simulink model "CC3"  (Simulink 7.5)
settings: Solver=ode45  StartTime=0.0  StopTime=300  RelTol=1e-3
settings Model: Creator=Fer  LastModifiedBy=Fer

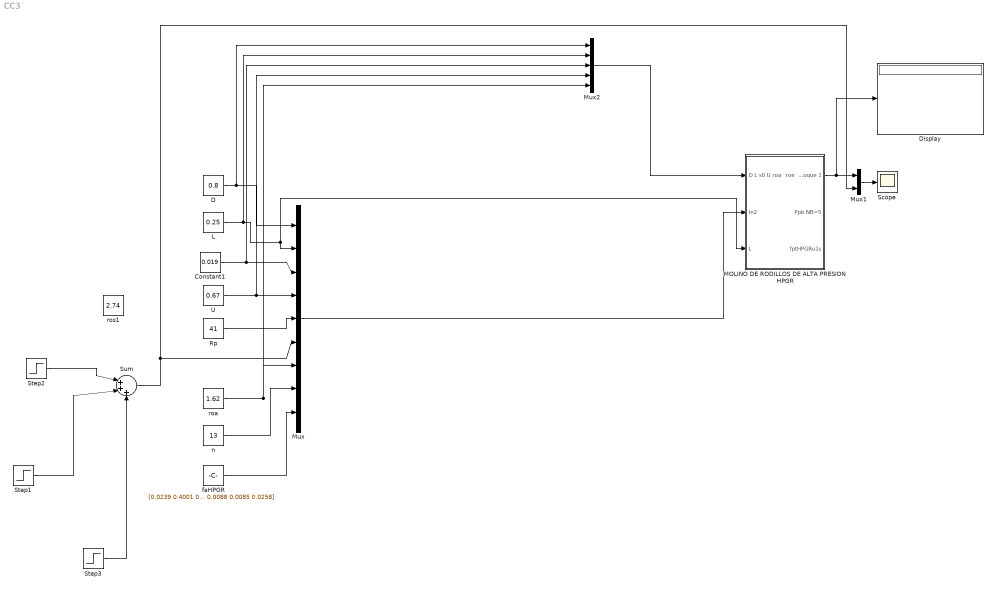
== system CC3 ==
  Constant1 : Constant  Value=0.019  OutDataType=fixdt(1, 16)  OutScaling=2^0
  D : Constant  Value=0.8  OutDataType=fixdt(1, 16)  OutScaling=2^0
  Display : Display
  L : Constant  Value=0.25  OutDataType=fixdt(1, 16)  OutScaling=2^0
  MOLINO DE RODILLOS DE ALTA PRESION HPGR : Subsystem
  Mux : Mux  Inputs=9
  Mux1 : Mux  Inputs=2
  Mux2 : Mux  Inputs=5
  Rp : Constant  Value=41  OutDataType=fixdt(1, 16)  OutScaling=2^0
  Scope : Scope
      settings: TimeRange=400  YMin=0  YMax=3  SaveName=ScopeData2
  Step1 : Step  Time=80  Before=3  After=7  SampleTime=0
  Step2 : Step  Time=80  Before=2.74  After=3  SampleTime=0
  Step3 : Step  Time=130  Before=3  SampleTime=0
  Sum : Sum  Inputs=|+++  OutDataType=fixdt(1, 16)  OutScaling=2^0
  U : Constant  Value=0.67  OutDataType=fixdt(1, 16)  OutScaling=2^0
  faHPGR : Constant  Value=[0.0239 0.4001 0.2089 0.1090 0.0549 0.0441 0.0542 0.0374 0.0159 0.0085 0.0088 0.0085 0.0258]  OutDataType=fixdt(1, 16)  OutScaling=2^0
  n : Constant  Value=13  OutDataType=fixdt(1, 16)  OutScaling=2^0
  roa : Constant  Value=1.62  OutDataType=fixdt(1, 16)  OutScaling=2^0
  ros1 : Constant  Value=2.74  OutDataType=fixdt(1, 16)  OutScaling=2^0
  wires:
  D/1 -> Mux/1, Mux2/1
  L/1 -> Mux/2, MOLINO DE RODILLOS DE ALTA PRESION HPGR/3(L), Mux2/2
  roa/1 -> Mux/7, Mux2/5
  n/1 -> Mux/8
  Mux/1 -> MOLINO DE RODILLOS DE ALTA PRESION HPGR/2(In2)
  Mux2/1 -> MOLINO DE RODILLOS DE ALTA PRESION HPGR/1(D L s0 U roa)
  faHPGR/1 -> Mux/9
  MOLINO DE RODILLOS DE ALTA PRESION HPGR/1(roe  bloque 1) -> Mux1/1, Display/1
  Mux1/1 -> Scope/1
  Step2/1 -> Sum/1
  Sum/1 -> Mux1/2, Mux/6
  Rp/1 -> Mux/5
  U/1 -> Mux/4, Mux2/4
  Step1/1 -> Sum/2
  Step3/1 -> Sum/3
  Constant1/1 -> Mux/3, Mux2/3

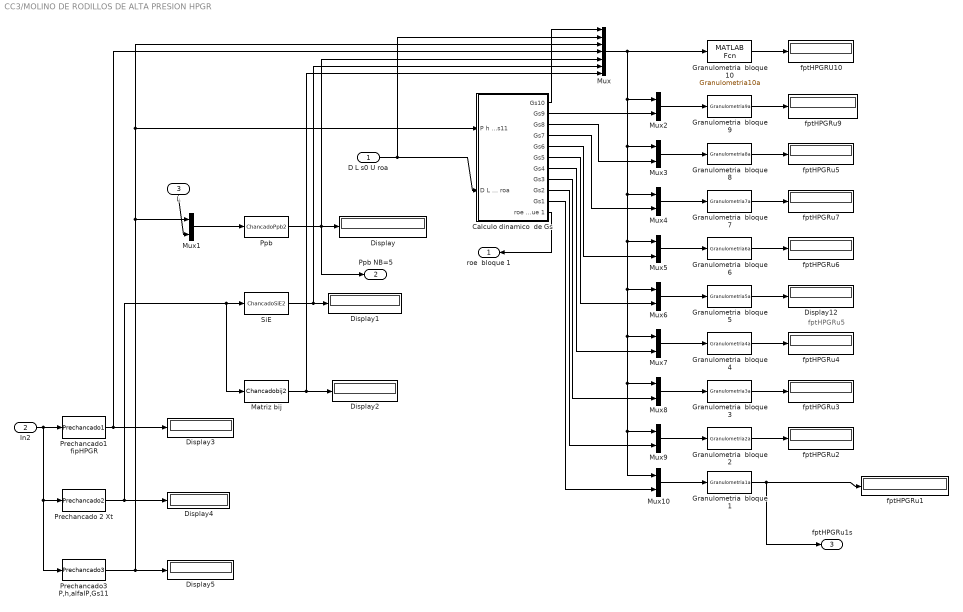
== system CC3/MOLINO DE RODILLOS DE ALTA PRESION HPGR ==
  note: fptHPGRu5
  D L s0 U roa : Inport
  In2 : Inport  Port=2
  L : Inport  Port=3
  Calculo dinamico  de Gs : Subsystem
  Display{,1..5,12} (7 alike) : Display
  Granulometria  bloque 1 : MATLABFcn  MATLABFcn=Granulometria1a
  Granulometria  bloque 10 : MATLABFcn  MATLABFcn=Granulometria10a
  Granulometria  bloque 2 : MATLABFcn  MATLABFcn=Granulometria2a
  Granulometria  bloque 3 : MATLABFcn  MATLABFcn=Granulometria3a
  Granulometria  bloque 4 : MATLABFcn  MATLABFcn=Granulometria4a
  Granulometria  bloque 5 : MATLABFcn  MATLABFcn=Granulometria5a
  Granulometria  bloque 6 : MATLABFcn  MATLABFcn=Granulometria6a
  Granulometria  bloque 7 : MATLABFcn  MATLABFcn=Granulometria7a
  Granulometria  bloque 8 : MATLABFcn  MATLABFcn=Granulometria8a
  Granulometria  bloque 9 : MATLABFcn  MATLABFcn=Granulometria9a
  Matriz bij : MATLABFcn  MATLABFcn=Chancadobij2
  Mux : Mux  Inputs=7
  Mux{1..10} (10 alike) : Mux  Inputs=2
  Ppb : MATLABFcn  MATLABFcn=ChancadoPpb2
  Prechancado 2 Xt : MATLABFcn  MATLABFcn=Prechancado2
  Prechancado1 fipHPGR : MATLABFcn  MATLABFcn=Prechancado1
  Prechancado3 P,h,alfaIP,Gs11 : MATLABFcn  MATLABFcn=Prechancado3
  SiE : MATLABFcn  MATLABFcn=ChancadoSiE2
  fptHPGRU10 : Display
  fptHPGRu{1..7,9} (8 alike) : Display
  roe  bloque 1 : Outport
  Ppb NB=5 : Outport  Port=2
  fptHPGRu1s : Outport  Port=3
  wires:
  Mux1/1 -> Ppb/1
  Ppb/1 -> Display/1, Ppb NB=5/1, Mux/5
  SiE/1 -> Display1/1, Mux/6
  Matriz bij/1 -> Display2/1, Mux/7
  L/1 -> Mux1/2
  D L s0 U roa/1 -> Calculo dinamico  de Gs/2(D L s0 U roa), Mux/2
  Calculo dinamico  de Gs/11(roe  bloque 1) -> roe  bloque 1/1
  Prechancado1 fipHPGR/1 -> Display3/1, Mux/4
  Prechancado 2 Xt/1 -> Display4/1, SiE/1, Matriz bij/1
  Prechancado3 P,h,alfaIP,Gs11/1 -> Display5/1, Mux1/1, Calculo dinamico  de Gs/1(P h alfaIP Gs11), Mux/3
  Calculo dinamico  de Gs/1(Gs10) -> Mux/1
  Mux/1 -> Granulometria  bloque 10/1, Mux2/1, Mux3/1, Mux4/1, Mux5/1, Mux6/1, Mux7/1, Mux8/1, Mux9/1, Mux10/1
  In2/1 -> Prechancado1 fipHPGR/1, Prechancado 2 Xt/1, Prechancado3 P,h,alfaIP,Gs11/1
  Granulometria  bloque 10/1 -> fptHPGRU10/1
  Calculo dinamico  de Gs/2(Gs9) -> Mux2/2
  Mux2/1 -> Granulometria  bloque 9/1
  Granulometria  bloque 9/1 -> fptHPGRu9/1
  Mux3/1 -> Granulometria  bloque 8/1
  Calculo dinamico  de Gs/3(Gs8) -> Mux3/2
  Calculo dinamico  de Gs/4(Gs7) -> Mux4/2
  Calculo dinamico  de Gs/5(Gs6) -> Mux5/2
  Mux4/1 -> Granulometria  bloque 7/1
  Mux5/1 -> Granulometria  bloque 6/1
  Granulometria  bloque 7/1 -> fptHPGRu7/1
  Granulometria  bloque 6/1 -> fptHPGRu6/1
  Calculo dinamico  de Gs/6(Gs5) -> Mux6/2
  Calculo dinamico  de Gs/7(Gs4) -> Mux7/2
  Calculo dinamico  de Gs/8(Gs3) -> Mux8/2
  Calculo dinamico  de Gs/9(Gs2) -> Mux9/2
  Calculo dinamico  de Gs/10(Gs1) -> Mux10/2
  Mux6/1 -> Granulometria  bloque 5/1
  Mux7/1 -> Granulometria  bloque 4/1
  Mux8/1 -> Granulometria  bloque 3/1
  Mux9/1 -> Granulometria  bloque 2/1
  Mux10/1 -> Granulometria  bloque 1/1
  Granulometria  bloque 5/1 -> Display12/1
  Granulometria  bloque 4/1 -> fptHPGRu4/1
  Granulometria  bloque 3/1 -> fptHPGRu3/1
  Granulometria  bloque 2/1 -> fptHPGRu2/1
  Granulometria  bloque 8/1 -> fptHPGRu5/1
  Granulometria  bloque 1/1 -> fptHPGRu1s/1, fptHPGRu1/1

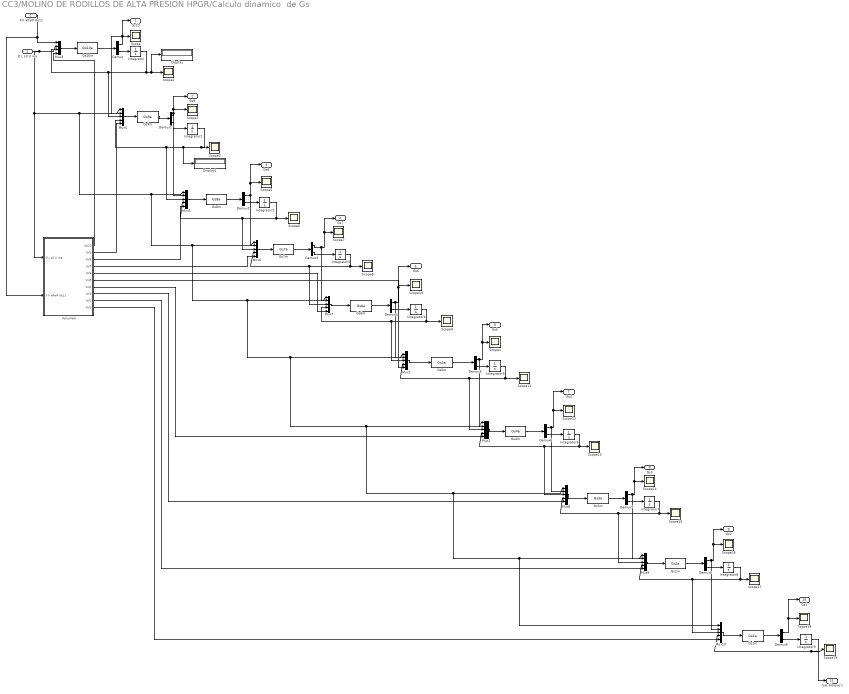
== system CC3/MOLINO DE RODILLOS DE ALTA PRESION HPGR/Calculo dinamico  de Gs ==
  P h alfaIP Gs11 : Inport
  D L s0 U roa : Inport  Port=2
  Demux{,1..9} (10 alike) : Demux  Outputs=2
  Display : Display
  Display1 : Display
  Gs10m : MATLABFcn  MATLABFcn=Gs10a
  Gs1m : MATLABFcn  MATLABFcn=Gs1a
  Gs2m : MATLABFcn  MATLABFcn=Gs2a
  Gs3m : MATLABFcn  MATLABFcn=Gs3a
  Gs4m : MATLABFcn  MATLABFcn=Gs4a
  Gs5m : MATLABFcn  MATLABFcn=Gs5a
  Gs6m : MATLABFcn  MATLABFcn=Gs6a
  Gs7m : MATLABFcn  MATLABFcn=Gs7a
  Gs8m : MATLABFcn  MATLABFcn=Gs8a
  Gs9m : MATLABFcn  MATLABFcn=Gs9a
  Integrator{,1..9} (10 alike) : Integrator  InitialCondition=1.6
  Mux{1..2,4..10} (9 alike) : Mux  Inputs=5
  Mux3 : Mux
  Scope{,1..19} (20 alike) : Scope
      Scope1 settings: SaveName=ScopeData10
      Scope10 settings: SaveName=ScopeData9
      Scope11 settings: SaveName=ScopeData11
      Scope12 settings: SaveName=ScopeData12
      Scope13 settings: SaveName=ScopeData13
      Scope14 settings: SaveName=ScopeData14
      Scope15 settings: SaveName=ScopeData15
      Scope16 settings: SaveName=ScopeData16
      Scope17 settings: SaveName=ScopeData17
      Scope18 settings: SaveName=ScopeData18
      Scope19 settings: SaveName=ScopeData19
      Scope3 settings: SaveName=ScopeData2
      Scope4 settings: SaveName=ScopeData3
      Scope5 settings: SaveName=ScopeData4
      Scope6 settings: SaveName=ScopeData5
      Scope7 settings: SaveName=ScopeData6
      Scope8 settings: SaveName=ScopeData7
      Scope9 settings: SaveName=ScopeData8
  Volumen : Subsystem
  Gs10 : Outport  OutDataType=fixdt(1, 16)  OutScaling=2^0
  Gs9 : Outport  Port=2  OutDataType=fixdt(1, 16)  OutScaling=2^0
  Gs8 : Outport  Port=3  OutDataType=fixdt(1, 16)  OutScaling=2^0
  Gs7 : Outport  Port=4  OutDataType=fixdt(1, 16)  OutScaling=2^0
  Gs6 : Outport  Port=5  OutDataType=fixdt(1, 16)  OutScaling=2^0
  Gs5 : Outport  Port=6  OutDataType=fixdt(1, 16)  OutScaling=2^0
  Gs4 : Outport  Port=7  OutDataType=fixdt(1, 16)  OutScaling=2^0
  Gs3 : Outport  Port=8  OutDataType=fixdt(1, 16)  OutScaling=2^0
  Gs2 : Outport  Port=9  OutDataType=fixdt(1, 16)  OutScaling=2^0
  Gs1 : Outport  Port=10  OutDataType=fixdt(1, 16)  OutScaling=2^0
  roe  bloque 1 : Outport  Port=11  OutDataType=fixdt(1, 16)  OutScaling=2^0
  wires:
  D L s0 U roa/1 -> Mux3/2, Mux6/1, Mux7/1, Mux1/1, Mux2/1, Mux8/1, Mux9/1, Mux10/1, Mux5/1, Mux4/1, Volumen/1(D L s0 U roa)
  Mux3/1 -> Gs10m/1
  Integrator/1 -> Mux3/3, Mux4/3, Scope4/1, Display/1
  Gs10m/1 -> Demux/1
  Demux/2 -> Integrator/1
  Demux/1 -> Scope/1, Mux4/2, Gs10/1
  Integrator1/1 -> Scope3/1, Mux4/4, Mux5/3, Display1/1
  Demux1/2 -> Integrator1/1
  Mux4/1 -> Gs9m/1
  Gs9m/1 -> Demux1/1
  Demux1/1 -> Mux5/2, Scope2/1, Gs9/1
  Mux5/1 -> Gs8m/1
  Gs8m/1 -> Demux2/1
  Demux2/2 -> Integrator2/1
  Integrator2/1 -> Mux5/4, Mux6/3, Scope6/1
  Demux2/1 -> Mux6/2, Scope5/1, Gs8/1
  Mux6/1 -> Gs7m/1
  Gs7m/1 -> Demux3/1
  Demux3/2 -> Integrator3/1
  Integrator3/1 -> Mux6/4, Mux7/3, Scope8/1
  Demux3/1 -> Mux7/2, Scope7/1, Gs7/1
  Mux7/1 -> Gs6m/1
  Gs6m/1 -> Demux4/1
  Demux4/2 -> Integrator4/1
  Integrator4/1 -> Mux7/4, Mux1/3, Scope9/1
  Demux4/1 -> Scope10/1, Gs6/1, Mux1/2
  P h alfaIP Gs11/1 -> Mux3/1, Volumen/2(P h alfaIP Gs11)
  Mux1/1 -> Gs5m/1
  Gs5m/1 -> Demux5/1
  Demux5/1 -> Scope1/1, Gs5/1, Mux2/2
  Demux5/2 -> Integrator5/1
  Integrator5/1 -> Mux1/4, Mux2/3, Scope11/1
  Mux2/1 -> Gs4m/1
  Gs4m/1 -> Demux6/1
  Demux6/2 -> Integrator6/1
  Demux6/1 -> Scope12/1, Gs4/1, Mux8/2
  Integrator6/1 -> Mux2/4, Mux8/3, Scope13/1
  Mux8/1 -> Gs3m/1
  Gs3m/1 -> Demux7/1
  Demux7/1 -> Scope14/1, Gs3/1, Mux9/2
  Demux7/2 -> Integrator7/1
  Integrator7/1 -> Mux8/4, Mux9/3, Scope15/1
  Gs2m/1 -> Demux8/1
  Demux8/1 -> Scope16/1, Gs2/1, Mux10/2
  Demux8/2 -> Integrator8/1
  Integrator8/1 -> Mux9/4, Mux10/3, Scope17/1
  Mux9/1 -> Gs2m/1
  Mux10/1 -> Gs1m/1
  Gs1m/1 -> Demux9/1
  Demux9/1 -> Gs1/1, Scope18/1
  Demux9/2 -> Integrator9/1
  Integrator9/1 -> Mux10/4, Scope19/1, roe  bloque 1/1
  Volumen/1(Vol10) -> Mux3/4
  Volumen/2(Vol9) -> Mux4/5
  Volumen/3(Vol8) -> Mux5/5
  Volumen/4(Vol7) -> Mux6/5
  Volumen/5(Vol6) -> Mux7/5
  Volumen/6(Vol5) -> Mux1/5
  Volumen/7(Vol4) -> Mux2/5
  Volumen/8(Vol3) -> Mux8/5
  Volumen/9(Vol2) -> Mux9/5
  Volumen/10(Vol1) -> Mux10/5

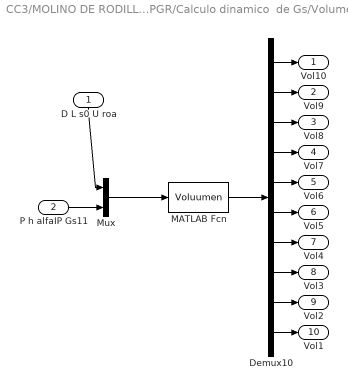
== system CC3/MOLINO DE RODILLOS DE ALTA PRESION HPGR/Calculo dinamico  de Gs/Volumen ==
  D L s0 U roa : Inport
  P h alfaIP Gs11 : Inport  Port=2
  Demux10 : Demux  Outputs=10
  MATLAB Fcn : MATLABFcn  MATLABFcn=Voluumen
  Mux : Mux  Inputs=2
  Vol10 : Outport
  Vol9 : Outport  Port=2
  Vol8 : Outport  Port=3
  Vol7 : Outport  Port=4
  Vol6 : Outport  Port=5
  Vol5 : Outport  Port=6
  Vol4 : Outport  Port=7
  Vol3 : Outport  Port=8
  Vol2 : Outport  Port=9
  Vol1 : Outport  Port=10
  wires:
  Mux/1 -> MATLAB Fcn/1
  MATLAB Fcn/1 -> Demux10/1
  D L s0 U roa/1 -> Mux/1
  P h alfaIP Gs11/1 -> Mux/2
  Demux10/1 -> Vol10/1
  Demux10/2 -> Vol9/1
  Demux10/3 -> Vol8/1
  Demux10/4 -> Vol7/1
  Demux10/5 -> Vol6/1
  Demux10/6 -> Vol5/1
  Demux10/7 -> Vol4/1
  Demux10/8 -> Vol3/1
  Demux10/9 -> Vol2/1
  Demux10/10 -> Vol1/1
